simulink library "VehDynaPlayGround"  (R2024b)
settings: Solver=VariableStepAuto  StartTime=0.0  StopTime=10.0  RelTol=1e-3
undefined symbols (not defined in the file or in its folder): A_F, C_af, C_ar, C_d, f, g, h_aero, h_gc, InitialX, InitialY, Iz, lf, lr, m, Nf, Nr, phi, r_stat, r_w, rho, theta, V_wind
libraries: slpidlib x5
(part 2 of 3)

== matlab function VehDynaPlayGround/Vehicle Dynamics/LateralDynamics/LateralDynamicWithNoise/LateralDynamicWithNoise ==
  data: dX output; X input; Vx input; dd input; phi_ref input; NoiseDdy input; NoiseDdpsi input; C_af parameter; C_ar parameter; lf parameter; lr parameter; Iz parameter; m parameter; g parameter
% ******************* Lateral dynamic controller *********************
%*********************************************************************
% Author: L.Arturo Torres-Romero
% Date: 22-10-2020
% BICYCLE MODEL OF LATERAL VEHICLE DYNAMICS
% Based on Rajamani chapter 2.3 page 30 and  in the next publication with
% the controller
% https://www.researchgate.net/publication/340166902_LATERAL_VEHICLE_DYNAMICS_AND_CONTROLLERS_DESIGN
%******************* PARAMETERS DESCRIPTIONS **********************
%******************************************************************
% m: vehicle mass
% g: gravity
% C_af : Cornering  stiffness  of  front  wheels.
% C_ar : Cornering  stiffness  of  rear  wheels.
% lf : distance fron the center of gravity to the front wheel axis.
% lr : distance fron the center of gravity to the rear wheel axis.
% Iz : this is the momentum of inertia of the vehicle respect the z axis.
% phi: is the road bank.
%******************************************************************
%******************* INPUTS DESCRIPTIONS **************************
%******************************************************************
% X:   (column vector)[y;dy;Psi;dPsi] states of the state space of 
%       the system that includes:
%      y  : Radius of the curve that the car is performing.
%      dy : Lateral velocity.
%      Psi  : Is the yaw angle respect to the inertial global system
%      dPsi : Angular velocity of the yaw angle.
% Vx: Logitudinal velocity.

function dX = DynamicBicycleModel2(X,Vx,dd, phi_ref, NoiseDdy, NoiseDdpsi, C_af, C_ar, lf, lr, Iz, m,g) % pd polos deseados
dX = [0;0;0;0];
y = X(1);
dy = X(2);
Psi = X(3);
dPsi = X(4);
phi = phi_ref;

theta_vf = atan((dy + lf*dPsi)/Vx);
theta_vr = atan((dy - lr*dPsi)/Vx);

alpha_f = dd - theta_vf; % lateral slip angle in front tires
alpha_r = -theta_vr; % lateral slip angle in rear tires

dX(1) = X(2);
dX(2) = NoiseDdy + (2*C_af*alpha_f + 2*C_ar*alpha_r)/m + g*sin(phi) - dPsi*Vx;
dX(3) = X(4);
dX(4) = NoiseDdpsi + (2*lf*C_af*alpha_f - 2*lr*C_ar*alpha_r)/Iz;

end

== matlab function VehDynaPlayGround/Control laws/LateralController/SMC_Conventional1 ==
  data: U output size=1; E input; Vx input; C_af parameter; g parameter; C_ar parameter; lf parameter; lr parameter; Iz parameter; m parameter
% ******************* Lateral dynamic controller *********************
%*********************************************************************
% Author: L.Arturo Torres-Romero
% Date: 22-10-2020
% This controller controlls the direction of a car, based in the dynamics
% described  in the next link and using the conventional sliding mode control 
% formulation with the procedure of converting to regular form: 
% https://www.researchgate.net/publication/340166902_LATERAL_VEHICLE_DYNAMICS_AND_CONTROLLERS_DESIGN
%******************* PARAMETERS DESCRIPTIONS **********************
%******************************************************************
% m: vehicle mass
% g: gravity
% C_af : Cornering  stiffness  of  front  wheels.
% C_ar : Cornering  stiffness  of  rear  wheels.
% lf : distance fron the center of gravity to the front wheel axis.
% lr : distance fron the center of gravity to the rear wheel axis.
% Iz : this is the momentum of inertia of the vehicle respect the z axis.
%******************************************************************
%******************* INPUTS DESCRIPTIONS **************************
%******************************************************************
% E:   (column vector)[e1;de1;e2;de2] states of the state space of 
%       the system that includes the errors as follows:
%      e1  : is the lateral position error respect the road.
%      de1 : derivative of e1.
%      e2  : is the yaw angle error with respect the road. 
%      de2 : derivarive of the e2.
% Vx: Logitudinal velocity.

%******************************************************************
% ******************* OUTPUTS DESCRIPTIONS ************************
%******************************************************************
% U: control coutput in radians. Angle of the frontal wheels respect to the
%    longitudinal axis
% isCtrl: when true means that the matrix Mc has full rank, and hence, the
%         system is controllable
%******************************************************************

function U = SMC_ConventionalCtrl(E, Vx, C_af, g, C_ar, lf, lr, Iz, m) % pd polos deseados
X = [0; 0; 0; 0];
X(1) = E(1);
X(2) = E(2);
X(3) = E(3);
X(4) = E(4);
n = 16;
lambda_1 = -1;
lambda_2 = -2;
%**************************************************
%******* Matrix A formulation *********************
A22 = -(2*C_af + 2*C_ar)/(m*Vx);
A23 = (2*C_af + 2*C_ar)/m;
A24 = (-2*C_af*lf + 2*C_ar*lr)/(m*Vx);
A42 = -(2*C_af*lf - 2*C_ar*lr)/(Iz*Vx);
A43 = (2*C_af*lf - 2*C_ar*lr)/Iz;
A44 = -(2*C_af*lf^2 + 2*C_ar*lr^2)/(Iz*Vx);

A = [0 1 0 0;0 A22 A23 A24;0 0 0 1;0 A42 A43 A44];
%**************************************************

%**************************************************
%******* Matrix B1 formulation ********************
B1_2 = 2*C_af/m;
B1_4 = 2*C_af*lf/Iz;

B1 = [0;B1_2;0;B1_4];
%***************************************************

%***************************************************
%******* Matrix B2 formulation *********************
B2_2 = -(2*C_af*lf - 2*C_ar*lr)/(m*Vx) - Vx;
B2_4 = -(2*C_af*lf^2 + 2*C_ar*lr^2)/(Iz*Vx);

B2 = [0;B2_2;0;B2_4];
%***************************************************


%***************************************************
%******* Matrix B3 formulation *********************
B3 = [0;g;0;0];
%***************************************************
x1 = X(1);
x2 = X(2);
x3 = X(3);
x4 = X(4);

%%%%%% this is with S2 = inv(B_2)
% sigma1 = -(lambda_2*x1 - x2 + lambda_2*x3)/B1_2;
% sigma2 = -(lambda_1*x1 - x4 + lambda_1*x3)/B1_4;
% u1 = -(A22*x2 + A23*x3 + A24*x4 - lambda_2*x2 - lambda_2*x4 + B1_2*n*sign(sigma1))/B1_2;
% u2 = -(A42*x2 + A43*x3 + A44*x4 - lambda_1*x2 - lambda_1*x4 + B1_4*n*sign(sigma2))/B1_4;


%%%%%% this is with S2 = eye(2)
sigma1 = -(abs(B1_4)*(lambda_1*x1 - x4 + lambda_1*x3))/B1_4;
sigma2 = -(abs(B1_2)*(lambda_2*x1 - x2 + lambda_2*x3))/B1_2;
u1 = -(A42*x2 + A43*x3 + A44*x4 - lambda_1*x2 - lambda_1*x4 + n*sign(B1_4)*sign(sigma1))/B1_4;
u2 = -(A22*x2 + A23*x3 + A24*x4 - lambda_2*x2 - lambda_2*x4 + n*sign(B1_2)*sign(sigma2))/B1_2;

ctrlVal =  (u2+u1)/2;

U = real(ctrlVal);    



%*****************************************************************************
%******* Live script for help in calculus of the controller ************
% 
% format rational
% syms A B Q R Tr B1_2 B1_4 A22 A23 A24 A42 A43 A44
% A = [0 1 0 0;0 A22 A23 A24;0 0 0 1;0 A42 A43 A44]
% B = [0 0;B1_2 0;0 0;0 B1_4]
% 
% [Q R] = qr(sym(B))
% 
% Tr= flipud(Q') % we need the cero part in the superior part
% rank(Tr)
% 
% B_ = Tr*B
% 
% A_ = Tr*A*inv(Tr)
% 
% % A_ matrix partition
% A_11 = A_(1:2,1:2)
% A_12 = A_(1:2,3:4)
% A_21 = A_(3:4,1:2)
% A_22 = A_(3:4,3:4)
% 
% syms M M11 M12 M21 M22 lambda_1 lambda_2
% M = [M11 M12;M21 M22];
% eqeigen = [lambda_1;lambda_2] == A_11 - A_12*M;
% H = solve(eqeigen,M);
% M_ = [H.M11 H.M12;H.M21 H.M22]
% 
% S2 = eye(2);
% %S2 = inv(B_(3:4,:))
% S = S2*[M_ eye(2)]*Tr;
% disp("surface S: ")
% expand(S)
% 
% syms n sigma_ x1 x2 x3 x4 u1 u2
% X = [x1;x2;x3;x4];
% U = [u1;u2];
% 
% SIGMA = S*X;
% Sigma_1 = simplify(SIGMA(1))
% Sigma_2 = simplify(SIGMA(2))
% 
% eqsolution = -n*sign(sigma_) == S*(A*X + B*U)
% sol1 = solve(eqsolution(1),u2);
% sol2 = solve(eqsolution(2),u1);
% 
% simplify(sol1)
% simplify(sol2)

== matlab function VehDynaPlayGround/Vehicle Dynamics/LateralDynamics/LateralDynamic ==
  data: dX output; X input; Vx input; dd input; C_af parameter; C_ar parameter; lf parameter; lr parameter; Iz parameter; m parameter; g parameter; phi_ref input
% ******************* Lateral dynamic controller *********************
%*********************************************************************
% Author: L.Arturo Torres-Romero
% Date: 22-10-2020
% BICYCLE MODEL OF LATERAL VEHICLE DYNAMICS
% Based on Rajamani chapter 2.3 page 30 and  in the next publication with
% the controller
% https://www.researchgate.net/publication/340166902_LATERAL_VEHICLE_DYNAMICS_AND_CONTROLLERS_DESIGN
%******************* PARAMETERS DESCRIPTIONS **********************
%******************************************************************
% m: vehicle mass
% g: gravity
% C_af : Cornering  stiffness  of  front  wheels.
% C_ar : Cornering  stiffness  of  rear  wheels.
% lf : distance fron the center of gravity to the front wheel axis.
% lr : distance fron the center of gravity to the rear wheel axis.
% Iz : this is the momentum of inertia of the vehicle respect the z axis.
% phi : is the road bank. not used in this model.
%******************************************************************
%******************* INPUTS DESCRIPTIONS **************************
%******************************************************************
% X:   (column vector)[y;dy;Psi;dPsi] states of the state space of 
%       the system that includes:
%      y  : Radius of the curve that the car is performing.
%      dy : Lateral velocity.
%      Psi  : Is the yaw angle respect to the inertial global system
%      dPsi : Angular velocity of the yaw angle.
% Vx: Logitudinal velocity.

function dX = DynamicBicycleModel(X,Vx,dd, C_af, C_ar, lf, lr, Iz, m,g, phi_ref) % pd polos deseados
dX = [0;0;0;0];
y = X(1);
dy = X(2);
Psi = X(3);
dPsi = X(4);
phi = phi_ref;

A22 = -(2*C_af+2*C_ar)/(m*Vx);
A24 = -Vx- (2*C_af*lf-2*C_ar*lr)/(m*Vx);
A42 = -(2*lf*C_af-2*lr*C_ar)/(Iz*Vx);
A44 = -(2*lf^2*C_af + 2*lr^2*C_ar)/(Iz*Vx);

B21 = 2*C_af/m;
B41 = 2*lf*C_af/Iz;

A = [0 1 0 0;0 A22 0 A24;0 0 0 1;0 A42 0 A44];
B = [0;B21;0;B41];

dX= A*X(1:4) + B*dd; 

end

== matlab function VehDynaPlayGround/Model helpers/CoordConvertRotation/MATLAB Function ==
  data: A input; B output; theta input
function B = RotateVector(A, theta)
B = [0;0];
R = [cos(theta) -sin(theta); sin(theta) cos(theta)];

B = R*A;

== matlab function VehDynaPlayGround/Vehicle Dynamics/LateralDynamics/LateralDynamic2 ==
  data: dX output; X input; Vx input; dd input; phi_ref input; C_af parameter; C_ar parameter; lf parameter; lr parameter; Iz parameter; m parameter; g parameter
% ******************* Lateral dynamic controller *********************
%*********************************************************************
% Author: L.Arturo Torres-Romero
% Date: 22-10-2020
% BICYCLE MODEL OF LATERAL VEHICLE DYNAMICS
% Based on Rajamani chapter 2.3 page 30 and  in the next publication with
% the controller
% https://www.researchgate.net/publication/340166902_LATERAL_VEHICLE_DYNAMICS_AND_CONTROLLERS_DESIGN
%******************* PARAMETERS DESCRIPTIONS **********************
%******************************************************************
% m: vehicle mass
% g: gravity
% C_af : Cornering  stiffness  of  front  wheels.
% C_ar : Cornering  stiffness  of  rear  wheels.
% lf : distance fron the center of gravity to the front wheel axis.
% lr : distance fron the center of gravity to the rear wheel axis.
% Iz : this is the momentum of inertia of the vehicle respect the z axis.
% phi: is the road bank.
%******************************************************************
%******************* INPUTS DESCRIPTIONS **************************
%******************************************************************
% X:   (column vector)[y;dy;Psi;dPsi] states of the state space of 
%       the system that includes:
%      y  : Radius of the curve that the car is performing.
%      dy : Lateral velocity.
%      Psi  : Is the yaw angle respect to the inertial global system
%      dPsi : Angular velocity of the yaw angle.
% Vx: Logitudinal velocity.

function dX = DynamicBicycleModel2(X,Vx,dd,phi_ref, C_af, C_ar, lf, lr, Iz, m,g) % pd polos deseados
dX = [0;0;0;0];
y = X(1);
dy = X(2);
Psi = X(3);
dPsi = X(4);

theta_vf = atan((dy + lf*dPsi)/Vx);
theta_vr = atan((dy - lr*dPsi)/Vx);

alpha_f = dd - theta_vf; % lateral slip angle in front tires
alpha_r = -theta_vr; % lateral slip angle in rear tires

dX(1) = X(2);
dX(2) = (2*C_af*alpha_f + 2*C_ar*alpha_r)/m + g*sin(phi_ref) - dPsi*Vx;
dX(3) = X(4);
dX(4) = (2*lf*C_af*alpha_f - 2*lr*C_ar*alpha_r)/Iz;

end

== matlab function VehDynaPlayGround/Electric Actuators/SteeringActuator/BLDC_AngleCtrl/Back EMF ==
  data: X input; Fabc output
function Fabc = fcn(X)
Fabc = [0;0;0];
    theta = mod(X(5),2*pi); %X(4)
    %theta = mod(X,2*pi);
    
    if (0<=theta)&&(theta<(pi/6))
        Fa = (6/pi)*theta;
    elseif ((pi/6)<=theta)&&(theta<(5*pi/6))
        Fa = 1;
    elseif ((5*pi/6<=theta))&&(theta<(7*pi/6))
        Fa = (6/pi)*(pi-theta);
    elseif ((7*pi/6)<=theta)&&(theta<(11*pi/6))
        Fa = -1;
    elseif ((11*pi/6)<=theta)&&(theta<(2*pi))
        Fa = (6/pi)*(theta-2*pi);
    else
        Fa = NaN;
    end
    
    if (0<=theta)&&(theta<(3*pi/6))
        Fb = -1;
    elseif ((3*pi/6)<=theta)&&(theta<(5*pi/6))
        Fb = (6/pi)*(theta-(2*pi)/3);
    elseif ((5*pi/6)<=theta)&&(theta<(9*pi/6))
        Fb = 1;
    elseif ((9*pi/6)<=theta)&&(theta<(11*pi/6))
        Fb = (6/pi)*(-theta+(5*pi)/3);
    elseif ((11*pi/6)<=theta)&&(theta<(2*pi))
        Fb = -1;
    else
        Fb = NaN;
    end
    
    if (0<=theta)&&(theta<(pi/6))
        Fc = 1;
    elseif ((pi/6)<=theta)&&(theta<(3*pi/6))
        Fc = (6/pi)*(pi/3-theta);
    elseif ((3*pi/6)<=theta)&&(theta<(7*pi/6))
        Fc = -1;
    elseif ((7*pi/6)<=theta)&&(theta<(9*pi/6))
        Fc = (6/pi)*(theta-(4*pi)/3);
    elseif ((9*pi/6)<=theta)&&(theta<(2*pi))
        Fc = 1;
    else
        Fc = NaN; 
    end
    
    
%     
     %Fa = sin(theta);
     %Fb = sin(theta - 2*pi/3);
     %Fc = sin(theta + 2*pi/3);
    
    Fabc = [Fa;Fb;Fc];
end

== matlab function VehDynaPlayGround/Electric Actuators/SteeringActuator/BLDC_AngleCtrl/InvParkClarke ==
  data: X_dq input; Y_abc output; theta input
function Y_abc = fcn(X_dq, theta)
X_dq0 = [X_dq; 0];

%inverse Park-Clarke power invariant
iT_PC = sqrt(2/3)*[cos(theta)          -sin(theta)            1/sqrt(2); ...
                  cos(theta-2*pi/3)   -sin(theta-2*pi/3)     1/sqrt(2); ...
                  cos(theta+2*pi/3)   -sin(theta+2*pi/3)     1/sqrt(2)];
%               
              
 %inverse Park-Clarke amplitude invariant
% iT_PC = [cos(theta)          -sin(theta)            1; ...
%          cos(theta-2*pi/3)   -sin(theta-2*pi/3)     1; ...
%          cos(theta+2*pi/3)   -sin(theta+2*pi/3)     1];



Y_abc =iT_PC*X_dq0;
end

== matlab function VehDynaPlayGround/Electric Actuators/SteeringActuator/BLDC_AngleCtrl/ParkClarke ==
  data: X_abc input; Y_dq output; theta input
function Y_dq = fcn(X_abc, theta)

% Park clarke transform eliminating the third element
PC_T = (sqrt(2)/2)*[sqrt(3)*cos(theta)  sin(theta)  -sin(theta) ; ...
                    -sqrt(3)*sin(theta)  cos(theta)  -cos(theta)];

Y_dq =PC_T*X_abc;
end

== matlab function VehDynaPlayGround/Control laws/LateralController/HOSMC_AckermanSuperTwist/HOSMC_AckermanSuperTwis1 ==
  data: U output size=1; E input; Vx input; Mu1 input; C_af parameter; g parameter; C_ar parameter; lf parameter; lr parameter; Iz parameter; m parameter; dMu1 output
% ******************* Lateral dynamic controller *********************
%*********************************************************************
% Author: L.Arturo Torres-Romero
% Date: 22-10-2020
% This controller controlls the direction of a car, based in the dynamics
% described  in the next link and using the conventional sliding mode control 
% formulation with the procedure of converting to regular form: 
% https://www.researchgate.net/publication/340166902_LATERAL_VEHICLE_DYNAMICS_AND_CONTROLLERS_DESIGN
%******************* PARAMETERS DESCRIPTIONS **********************
%******************************************************************
% m: vehicle mass
% g: gravity
% C_af : Cornering  stiffness  of  front  wheels.
% C_ar : Cornering  stiffness  of  rear  wheels.
% lf : distance fron the center of gravity to the front wheel axis.
% lr : distance fron the center of gravity to the rear wheel axis.
% Iz : this is the momentum of inertia of the vehicle respect the z axis.
%******************************************************************
%******************* INPUTS DESCRIPTIONS **************************
%******************************************************************
% E:   (column vector)[e1;de1;e2;de2] states of the state space of 
%       the system that includes the errors as follows:
%      e1  : is the lateral position error respect the road.
%      de1 : derivative of e1.
%      e2  : is the yaw angle error with respect the road. 
%      de2 : derivarive of the e2.
% Vx: Logitudinal velocity.

%******************************************************************
% ******************* OUTPUTS DESCRIPTIONS ************************
%******************************************************************
% U: control coutput in radians. Angle of the frontal wheels respect to the
%    longitudinal axis
% isCtrl: when true means that the matrix Mc has full rank, and hence, the
%         system is controllable
%******************************************************************

function [U, dMu1] = SMC_AckermanSuperTwistingCtrl(E, Vx, Mu1,C_af, g, C_ar, lf, lr, Iz, m) % pd polos deseados
X = [0; 0; 0; 0];
X(1) = E(1);
X(2) = E(2);
X(3) = E(3);
X(4) = E(4);
%**************************************************
%******* Matrix A formulation *********************
A22 = -(2*C_af + 2*C_ar)/(m*Vx);
A23 = (2*C_af + 2*C_ar)/m;
A24 = (-2*C_af*lf + 2*C_ar*lr)/(m*Vx);
A42 = -(2*C_af*lf - 2*C_ar*lr)/(Iz*Vx);
A43 = (2*C_af*lf - 2*C_ar*lr)/Iz;
A44 = -(2*C_af*lf^2 + 2*C_ar*lr^2)/(Iz*Vx);

A = [0 1 0 0;0 A22 A23 A24;0 0 0 1;0 A42 A43 A44];
%**************************************************

%**************************************************
%******* Matrix B1 formulation ********************
B1_2 = 2*C_af/m;
B1_4 = 2*C_af*lf/Iz;

B1 = [0;B1_2;0;B1_4];
%***************************************************

%***************************************************
%******* Matrix B2 formulation *********************
B2_2 = -(2*C_af*lf - 2*C_ar*lr)/(m*Vx) - Vx;
B2_4 = -(2*C_af*lf^2 + 2*C_ar*lr^2)/(Iz*Vx);

B2 = [0;B2_2;0;B2_4];
%***************************************************


%***************************************************
%******* Matrix B3 formulation *********************
B3 = [0;g;0;0];
%***************************************************


%***************************************************
%******* Verification of controllability and output 
% calculation of the controller
%**************************************************
d_k = 0;
Mc = [B1 A*B1 A^2*B1 A^3*B1];
rankVal = rank(Mc);
    if rankVal < size(A,1)
        %disp('Not completely state controllable');
        isCtrl = 0;
        d_k = 0;
    else
        %disp('Completely state controllable');
        isCtrl = 1;
        % Pole placement
        %Pd =[-5-3i -5+3i -7 -10];
        Pd =[-5-5i -5+5i -7 -10];

        H = (A- Pd(1)*eye(4)) * (A- Pd(2)*eye(4)) * (A- Pd(3)*eye(4)) * (A- Pd(4)*eye(4));

        %ackerman formula
        K = [0 0 0 1]*Mc^-1*H;
        d_k = -K*X;  
    end

%*********** Controller parameters **************
k_smc = 100;   %10
sigma = 40;    %60
gamma1 = 1;
gamma2 = 1;
gamma = [0 gamma1 0 gamma2];

h_c = gamma*[0;3;0;3];
g_c = gamma*B1;
q = 0.3;

UM = abs(h_c/g_c)/q;

%***********************************************
e_c = gamma*[0; X(1);0;X(3)];
d_u = (-1/(gamma*B1))*(sigma*sqrt(abs(e_c))*sign(e_c) + Mu1);

if abs(Mu1) > UM 
   dMu1 = -Mu1;
else
   dMu1 = -k_smc*sign(e_c); 
end

ctrlVal = d_k + d_u;

U = real(ctrlVal);

== matlab function VehDynaPlayGround/Control laws/LateralController/SMC_Conventional2 ==
  data: U output size=1; E input; Vx input; dPsi_des input; C_af parameter; g parameter; C_ar parameter; lf parameter; lr parameter; Iz parameter; m parameter; phi_ref input

% ******************* Lateral dynamic controller *********************
%*********************************************************************
% Author: L.Arturo Torres-Romero
% Date: 22-10-2020
% This controller controlls the direction of a car, based in the dynamics
% described  in the next link and using the conventional sliding mode control 
% formulation with the procedure of converting to regular form: 
% https://www.researchgate.net/publication/340166902_LATERAL_VEHICLE_DYNAMICS_AND_CONTROLLERS_DESIGN
%******************* PARAMETERS DESCRIPTIONS **********************
%******************************************************************
% m: vehicle mass
% g: gravity
% C_af : Cornering  stiffness  of  front  wheels.
% C_ar : Cornering  stiffness  of  rear  wheels.
% lf : distance fron the center of gravity to the front wheel axis.
% lr : distance fron the center of gravity to the rear wheel axis.
% Iz : this is the momentum of inertia of the vehicle respect the z axis.
%******************************************************************
%******************* INPUTS DESCRIPTIONS **************************
%******************************************************************
% E:   (column vector)[e1;de1;e2;de2] states of the state space of 
%       the system that includes the errors as follows:
%      e1  : is the lateral position error respect the road.
%      de1 : derivative of e1.
%      e2  : is the yaw angle error with respect the road. 
%      de2 : derivarive of the e2.
% Vx: Logitudinal velocity.

%******************************************************************
% ******************* OUTPUTS DESCRIPTIONS ************************
%******************************************************************
% U: control coutput in radians. Angle of the frontal wheels respect to the
%    longitudinal axis
% isCtrl: when true means that the matrix Mc has full rank, and hence, the
%         system is controllable
%******************************************************************

function U = SMC_ConventionalCtr2(E, Vx, dPsi_des,C_af, g, C_ar, lf, lr, Iz, m, phi_ref) % pd polos deseados
J = [0; 0; 0; 0];
J(1) = E(3);
J(2) = E(4);
J(3) = E(1);
J(4) = E(2);
phi = phi_ref;
%**************************************************
%******* Matrix A formulation *********************
A22 = -(2*C_af + 2*C_ar)/(m*Vx);
A23 = (2*C_af + 2*C_ar)/m;
A24 = (-2*C_af*lf + 2*C_ar*lr)/(m*Vx);
A42 = -(2*C_af*lf - 2*C_ar*lr)/(Iz*Vx);
A43 = (2*C_af*lf - 2*C_ar*lr)/Iz;
A44 = -(2*C_af*lf^2 + 2*C_ar*lr^2)/(Iz*Vx);

%A = [0 1 0 0;0 A22 A23 A24;0 0 0 1;0 A42 A43 A44];
A = [0 0 0 1;0 A42 A43 A44;0 1 0 0;0 A22 A23 A24];

%**************************************************

%**************************************************
%******* Matrix B1 formulation ********************
B1_2 = 2*C_af/m;
B1_4 = 2*C_af*lf/Iz;

%B1 = [0;B1_2;0;B1_4];
B1 = [0;B1_4;0;B1_2];
%***************************************************

%***************************************************
%******* Matrix B2 formulation *********************
B2_2 = -(2*C_af*lf - 2*C_ar*lr)/(m*Vx) - Vx;
B2_4 = -(2*C_af*lf^2 + 2*C_ar*lr^2)/(Iz*Vx);

B2 = [0;B2_4;0;B2_2];
%***************************************************


%***************************************************
%******* Matrix B3 formulation *********************
B3 = [0;g;0;0];
%***************************************************

l1 = (A24 - Vx)*dPsi_des +g*sin(phi);
l2 = A44*dPsi_des;
L = [0;l2;0;l1];

C = [B1 A*B1 A^2*B1 A^3*B1]; % controllability matrix
Cinv = inv(C);
q = Cinv(4,:);
P = [q;q*A;q*A^2;q*A^3];
Tr = P;

X = Tr*J;

%%%%%%%%%%%%%%%%%%%%%%%%%%%%% SMC settings %%%%%%%%%%%%%%%%%%%%%%%%%%%%%%%
n1 = 140000;
lambda_1 = -2;
lambda_2 = -7;
lambda_3 = -3;

S = [(1000000*lambda_1*lambda_2*lambda_3)/(A23*B1_4 - A43*B1_2), (1000000*(A23^2*B1_4^3 + A43^2*B1_2^2*B1_4 + A22*A23*A24*B1_4^3 - A42*A43*A44*B1_2^3 - 2*A23*A43*B1_2*B1_4^2 - A43*A44*B1_2^3*lambda_1 - A43*A44*B1_2^3*lambda_2 - A43*A44*B1_2^3*lambda_3 - A22*A23*A44*B1_2*B1_4^2 - A22*A24*A43*B1_2*B1_4^2 - A23*A24*A42*B1_2*B1_4^2 + A22*A43*A44*B1_2^2*B1_4 + A23*A42*A44*B1_2^2*B1_4 + A24*A42*A43*B1_2^2*B1_4 - A23*A24*B1_2*B1_4^2*lambda_1 - A23*A24*B1_2*B1_4^2*lambda_2 - A23*A24*B1_2*B1_4^2*lambda_3 + A23*A44*B1_2^2*B1_4*lambda_1 + A24*A43*B1_2^2*B1_4*lambda_1 + A23*A44*B1_2^2*B1_4*lambda_2 + A24*A43*B1_2^2*B1_4*lambda_2 + A23*A44*B1_2^2*B1_4*lambda_3 + A24*A43*B1_2^2*B1_4*lambda_3 - A23*B1_2*B1_4^2*lambda_1*lambda_2 - A23*B1_2*B1_4^2*lambda_1*lambda_3 - A23*B1_2*B1_4^2*lambda_2*lambda_3 + A43*B1_2^2*B1_4*lambda_1*lambda_2 + A43*B1_2^2*B1_4*lambda_1*lambda_3 + A43*B1_2^2*B1_4*lambda_2*lambda_3 - A44*B1_2^3*lambda_1*lambda_2*lambda_3 + A22*B1_2*B1_4^2*lambda_1*lambda_2*lambda_3 + A24*B1_2^2*B1_4*lambda_1*lambda_2*lambda_3 - A42*B1_2^2*B1_4*lambda_1*lambda_2*lambda_3))/((A23*B1_4 - A43*B1_2)*(A24^2*B1_2*B1_4^2 - 2*A24*A44*B1_2^2*B1_4 - A42*A24*B1_2*B1_4^2 + A22*A24*B1_4^3 + A44^2*B1_2^3 + A42*A44*B1_2^2*B1_4 - A22*A44*B1_2*B1_4^2 - A43*B1_2*B1_4^2 + A23*B1_4^3)), (1000000*(A23^2*B1_4^3*lambda_1 + A23^2*B1_4^3*lambda_2 + A23^2*B1_4^3*lambda_3 + A23^2*A24*B1_4^3 - A43^2*A44*B1_2^3 + A24*A43^2*B1_2^2*B1_4 - A23^2*A44*B1_2*B1_4^2 + A43^2*B1_2^2*B1_4*lambda_1 + A43^2*B1_2^2*B1_4*lambda_2 + A43^2*B1_2^2*B1_4*lambda_3 - 2*A23*A24*A43*B1_2*B1_4^2 + 2*A23*A43*A44*B1_2^2*B1_4 - 2*A23*A43*B1_2*B1_4^2*lambda_1 - 2*A23*A43*B1_2*B1_4^2*lambda_2 - 2*A23*A43*B1_2*B1_4^2*lambda_3 - A22*A23*B1_4^3*lambda_1*lambda_2 - A22*A23*B1_4^3*lambda_1*lambda_3 - A22*A23*B1_4^3*lambda_2*lambda_3 - A43*A44*B1_2^3*lambda_1*lambda_2 - A43*A44*B1_2^3*lambda_1*lambda_3 - A43*A44*B1_2^3*lambda_2*lambda_3 + A22^2*B1_4^3*lambda_1*lambda_2*lambda_3 + A42^2*B1_2^2*B1_4*lambda_1*lambda_2*lambda_3 - A23*A24*B1_2*B1_4^2*lambda_1*lambda_2 - A23*A24*B1_2*B1_4^2*lambda_1*lambda_3 - A23*A24*B1_2*B1_4^2*lambda_2*lambda_3 + A22*A43*B1_2*B1_4^2*lambda_1*lambda_2 + A23*A42*B1_2*B1_4^2*lambda_1*lambda_2 + A22*A43*B1_2*B1_4^2*lambda_1*lambda_3 + A23*A42*B1_2*B1_4^2*lambda_1*lambda_3 + A22*A43*B1_2*B1_4^2*lambda_2*lambda_3 + A23*A42*B1_2*B1_4^2*lambda_2*lambda_3 + A23*A44*B1_2^2*B1_4*lambda_1*lambda_2 + A24*A43*B1_2^2*B1_4*lambda_1*lambda_2 + A23*A44*B1_2^2*B1_4*lambda_1*lambda_3 + A24*A43*B1_2^2*B1_4*lambda_1*lambda_3 + A23*A44*B1_2^2*B1_4*lambda_2*lambda_3 + A24*A43*B1_2^2*B1_4*lambda_2*lambda_3 - A42*A43*B1_2^2*B1_4*lambda_1*lambda_2 - A42*A43*B1_2^2*B1_4*lambda_1*lambda_3 - A42*A43*B1_2^2*B1_4*lambda_2*lambda_3 + A42*A44*B1_2^3*lambda_1*lambda_2*lambda_3 - A23*B1_2*B1_4^2*lambda_1*lambda_2*lambda_3 + A43*B1_2^2*B1_4*lambda_1*lambda_2*lambda_3 + A22*A24*B1_2*B1_4^2*lambda_1*lambda_2*lambda_3 - 2*A22*A42*B1_2*B1_4^2*lambda_1*lambda_2*lambda_3 - A22*A44*B1_2^2*B1_4*lambda_1*lambda_2*lambda_3 - A24*A42*B1_2^2*B1_4*lambda_1*lambda_2*lambda_3))/((A23*B1_4 - A43*B1_2)*(A24^2*B1_2*B1_4^2 - 2*A24*A44*B1_2^2*B1_4 - A42*A24*B1_2*B1_4^2 + A22*A24*B1_4^3 + A44^2*B1_2^3 + A42*A44*B1_2^2*B1_4 - A22*A44*B1_2*B1_4^2 - A43*B1_2*B1_4^2 + A23*B1_4^3)), (1000000*(A23*A24^2*B1_4^3 - A43*A44^2*B1_2^3 + A23*B1_4^3*lambda_1*lambda_2 + A23*B1_4^3*lambda_1*lambda_3 + A23*B1_4^3*lambda_2*lambda_3 + A23*A44^2*B1_2^2*B1_4 - A24^2*A43*B1_2*B1_4^2 + A23*A24*B1_4^3*lambda_1 + A23*A24*B1_4^3*lambda_2 + A23*A24*B1_4^3*lambda_3 - 2*A23*A24*A44*B1_2*B1_4^2 + 2*A24*A43*A44*B1_2^2*B1_4 - A23*A44*B1_2*B1_4^2*lambda_1 - A24*A43*B1_2*B1_4^2*lambda_1 - A23*A44*B1_2*B1_4^2*lambda_2 - A24*A43*B1_2*B1_4^2*lambda_2 - A23*A44*B1_2*B1_4^2*lambda_3 - A24*A43*B1_2*B1_4^2*lambda_3 + A43*A44*B1_2^2*B1_4*lambda_1 + A43*A44*B1_2^2*B1_4*lambda_2 + A43*A44*B1_2^2*B1_4*lambda_3 - A43*B1_2*B1_4^2*lambda_1*lambda_2 - A43*B1_2*B1_4^2*lambda_1*lambda_3 - A43*B1_2*B1_4^2*lambda_2*lambda_3 - A22*B1_4^3*lambda_1*lambda_2*lambda_3 - A24*B1_2*B1_4^2*lambda_1*lambda_2*lambda_3 + A42*B1_2*B1_4^2*lambda_1*lambda_2*lambda_3 + A44*B1_2^2*B1_4*lambda_1*lambda_2*lambda_3))/((A23*B1_4 - A43*B1_2)*(A24^2*B1_2*B1_4^2 - 2*A24*A44*B1_2^2*B1_4 - A42*A24*B1_2*B1_4^2 + A22*A24*B1_4^3 + A44^2*B1_2^3 + A42*A44*B1_2^2*B1_4 - A22*A44*B1_2*B1_4^2 - A43*B1_2*B1_4^2 + A23*B1_4^3))];

%%%%%%%%%%%%%%%%%%%%%%%%%%%%%%%%%%%%%%%%%%%%%%%%%%%%%%%%%%%%%%%%%%%%%%%%%%%%

sigma1 = S*X;
ctrlVal = -(S*B1)\(n1*sign(sigma1)+ S*A*X +S*L);
U = real(ctrlVal);    



%*****************************************************************************
%******* Live script for help in calculus of the controller ************
% 
% format rational
% syms A B Q R Tr B1_2 B1_4 A22 A23 A24 A42 A43 A44 delta x1 x2 x3 x4 l1 l2
% 
% % X  = [x1;x2;x3;x4]
% % A  = [0 1 0 0;0 A22 A23 A24;0 0 0 1;0 A42 A43 A44]
% % B1 = [0;B1_2;0;B1_4]
% % L  = [0;l1;0;l2]
% 
% X  = [x3;x4;x1;x2]
% A  = [0 0 0 1;0 A42 A43 A44;0 1 0 0;0 A22 A23 A24]
% B1 = [0;B1_4;0;B1_2]
% L  = [0;l2;0;l1]
% 
% %%%%%%%%%%%%%%%% Transform (Tr) with ackerman form %%%%%%%%%%%%%%%%
% % C = [B1 A*B1 A^2*B1 A^3*B1] % controllability matrix
% % tmp1 = [0 0 0 1]/C;
% % Tr=[tmp1;tmp1*A;tmp1*A^2;tmp1*A^3] % state transformation
% % disp("tmp1")
% % size(tmp1)
% % disp("tmp1*A")
% % size(tmp1*A)
% % disp("tmp1*A^2")
% % size(tmp1*A^2)
% % disp("tmp1*A^3")
% % size(tmp1*A^3)
% % disp("C:")
% % size(C)
% % disp("tmp1:")
% % size(tmp1)
% % disp("Tr:")
% % size(Tr)
% %%%%%%%%%%%%%%%%%%%%%%%%%%%%%%%%%%%%%%%%%%%%%%%%%%%%%%%%%%%%%%%%%
% 
% %%%%%%%%%%%% Transform (Tr) with Utkin apprach %%%%%%%%%%%%%%%%%%
% % B_1 = [0;0;B1_4];
% % B_2 = B1_2;
% % 
% % a = eye(3)
% % b = -B_1*(B_2^(-1))
% % c = [0 0 0]
% % d = B_2^(-1)
% % 
% % Tr = [a b;c d];
% %%%%%%%%%%%%%%%%%%%%%%%%%%%%%%%%%%%%%%%%%%%%%%%%%%%%%%%%%%%%%%%%%%
% 
% 
% %%%%%%%%%%%%%%%% Transform (Tr) with linear system controller form %%%%%%%%%%%%%%%%
% C = [B1 A*B1 A^2*B1 A^3*B1] % controllability matrix
% Cinv = inv(C)
% q = Cinv(4,:)
% P = [q;q*A;q*A^2;q*A^3]
% Tr = P
% %%%%%%%%%%%%%%%%%%%%%%%%%%%%%%%%%%%%%%%%%%%%%%%%%%%%%%%%%%
% 
% A_ = simplify(Tr*A/Tr)
% B_ = simplify(Tr*B1)
% 
% A_11 = A_(1:3,1:3);
% A_12 = A_(1:3,4);
% 
% syms s1 s2 s3 lambda lambda_1 lambda_2 lambda_3 S2
% 
% %find paramters given eigenvalues
% S = [s1 s2 s3];
% eqeigen = det(lambda*eye(3) - (A_11 - A_12*S));
% eqeigen = simplify(eqeigen);
% eqeigen = collect(eqeigen,lambda);
% polyCoef = coeffs(eqeigen, lambda);
% polyCoef = fliplr(polyCoef)
% %%%%%%%%%%%%%%%
% % desired polinomial characteristic
% desiredPoly = (lambda + lambda_1)*(lambda + lambda_2)*(lambda + lambda_3);
% desiredPoly = collect(desiredPoly);
% desiredCoefs = coeffs(desiredPoly, lambda);
% desiredCoefs = fliplr(desiredCoefs)
% 
% eq1 = desiredCoefs(1) == polyCoef(1);
% eq2 = desiredCoefs(2) == polyCoef(2);
% eq3 = desiredCoefs(3) == polyCoef(3);
% eq4 = desiredCoefs(4) == polyCoef(4);
% 
% system1 = [eq2;eq3;eq4];
% sol = solve(system1,[s1 s2 s3]);
% S_ = [sol.s1 sol.s2 sol.s3]
% 
% %test eigen values:
% charEq1 = subs(eqeigen,s1,sol.s1);
% charEq2 = subs(charEq1,s2,sol.s2);
% charEq3 = subs(charEq2,s3,sol.s3)
% tf = isAlways(charEq3==desiredPoly)
% 
% S2 = 1000000;
% S = S2*[S_ 1]*Tr;
% %S = [S_ 1]*Tr;
% disp("!!!!!!!!surface S: ")
% simplify(S)
% 
% 
% syms n sigma1 x1 x2 x3 x4 u1 u2 n1 n2 
% X = [x1;x2;x3;x4];
% U = u1;
% 
% SIGMA = S*X;
% 
% % rewriting to the original forms %%%%%%%%%%%%%%%
% X  = [x1;x2;x3;x4]
% A  = [0 1 0 0;0 A22 A23 A24;0 0 0 1;0 A42 A43 A44]
% B1 = [0;B1_2;0;B1_4]
% %%%%%%%%%%%%%%%%%%%%%%%%%%%%%%%%%%%%%%%%%%%%%%%
% 
% 
% disp("!!!!! Sliding function sigma_1: ")
% Sigma_1 = simplify(SIGMA);
% Sigma_1 = collect(Sigma_1,[x1;x2;x3;x4])
% 
% eqsolution = -n1*sign(sigma1) == S*(A*X + B1*U +L);
% sol1 = solve(eqsolution,u1);
% 
% disp("!!!!! final control u: ")
% finalControl = simplify(sol1);
% finalControl = collect(finalControl,[x1;x2;x3;x4])
% 
% 
% U = -inv(S*B1)*(n1*sign(sigma1)+ S*A*X +S*L)
% 
% isAlways(finalControl==U)

== matlab function VehDynaPlayGround/Tires/Tyre ModelV1/MagicFormula ==
  data: X input; Y output; F_zf input
%BASED ON
%Massimo Guiggiani, The Science of Vehicle Dynamics, Pisa, Italy, Springer Netherlands, 2014.
%Chapter 2.12
%The values of the MF were obtained from the graph in fig. 2.22
function Y = XTireForce(X, F_zf) 
% B stiffness factor
% C shape factor
% D peak value
% E curvature factor
% Sh horizontal shift
% Sv vertical shift

Sh = 0;% Sh horizontal shift
Sv = 0; %vertical shift

D = 3; % ym, maximum value Experimental from graph
C = 1.5;
B = 20;
E = 0;

x = X-Sh;
gamma = C*atan(B*x-E*(B*x-atan(B*x)));
y = F_zf*D*sin(gamma);
Y = (y - Sv);

== matlab function VehDynaPlayGround/Control laws/LateralController/HOSMC_BlocksSuperTwisting/HOSMC_SuperTwisting ==
  data: U output size=1; E input; Vx input; dPsi_des input; phi_ref input; v input; C_af parameter; g parameter; C_ar parameter; lf parameter; lr parameter; Iz parameter; m parameter; dv output; d_u output
% ******************* Lateral dynamic controller *********************

%*********************************************************************
% Author: L.Arturo Torres-Romero
% Date: 22-10-2020
% This controller controlls the direction of a car, based in the dynamics
% described  in the next link and using the conventional sliding mode control 
% formulation with the procedure of converting to regular form: 
% https://www.researchgate.net/publication/340166902_LATERAL_VEHICLE_DYNAMICS_AND_CONTROLLERS_DESIGN
%******************* PARAMETERS DESCRIPTIONS **********************
%******************************************************************
% m: vehicle mass
% g: gravity
% C_af : Cornering  stiffness  of  front  wheels.
% C_ar : Cornering  stiffness  of  rear  wheels.
% lf : distance fron the center of gravity to the front wheel axis.
% lr : distance fron the center of gravity to the rear wheel axis.
% Iz : this is the momentum of inertia of the vehicle respect the z axis.
%******************************************************************
%******************* INPUTS DESCRIPTIONS **************************
%******************************************************************
% E:   (column vector)[e1;de1;e2;de2] states of the state space of 
%       the system that includes the errors as follows:
%      e1  : is the lateral position error respect the road.
%      de1 : derivative of e1.
%      e2  : is the yaw angle error with respect the road. 
%      de2 : derivarive of the e2.
% Vx: Logitudinal velocity.

%******************************************************************
% ******************* OUTPUTS DESCRIPTIONS ************************
%******************************************************************
% U: control coutput in radians. Angle of the frontal wheels respect to the
%    longitudinal axis
% isCtrl: when true means that the matrix Mc has full rank, and hence, the
%         system is controllable
%******************************************************************

function [U, dv,d_u] = HOSMC_SuperTwistingCtrl(E, Vx,dPsi_des, phi_ref, v,C_af, g, C_ar, lf, lr, Iz, m) % pd polos deseados
Y1 = [0;0];
Y2 = [0;0];

Y1 = [E(1);E(3)];
Y2 = [E(2);E(4)];
e = [E(2);E(3);E(4)];
phi = phi_ref;

%**************************************************
%******* Matrix A formulation *********************
A22 = -(2*C_af + 2*C_ar)/(m*Vx);
A23 = (2*C_af + 2*C_ar)/m;
A24 = (-2*C_af*lf + 2*C_ar*lr)/(m*Vx);
A42 = -(2*C_af*lf - 2*C_ar*lr)/(Iz*Vx);
A43 = (2*C_af*lf - 2*C_ar*lr)/Iz;
A44 = -(2*C_af*lf^2 + 2*C_ar*lr^2)/(Iz*Vx);

A = [A22 A23 A24;A42 A43 A44];

%**************************************************
%******* Matrix B1 formulation ********************
B1_2 = 2*C_af/m;
B1_4 = 2*C_af*lf/Iz;

B1 = [B1_2;B1_4];
%***************************************************

%***************************************************
%******* Matrix L formulation *********************
l1 = (A24 - Vx)*dPsi_des +g*sin(phi);
l2 = A44*dPsi_des;
L = [l1;l2];

%***************************************************

%%
%%%%%%%%%%%%%% SUPER TWISTING 1 %%%%%%%%%%%%%%%%%
% %*********** Controller parameters **************
k1 = 7;%6;      %7   18
k2 = 18;%8;
%sigma = 10;    %60   10
gamma1 = 1;
gamma2 = 0.9;
gamma = [gamma1 gamma2];
%***************************************
h_c = abs(gamma*[0.8;0.4]);
g_c = abs(gamma*B1);
U_M = pi/16;

q = abs(h_c/g_c)/U_M + 0.01;
C = abs(h_c)+ 0.5;
k_v = C/(gamma*B1) + 3; %k_v = C/(gamma*B1) + 0.5;

k_u = sqrt(2/(gamma*B1*k_v - C));
k_u = k_u*(gamma*B1*k_v + C)*(1+q);
k_u = k_u/((gamma*B1)*(1-q)) + 1; %k_u = k_u/((gamma*B1)*(1-q)) + 0.8;



%***********************************************
e_b = -gamma*(k1*Y1+Y2);
d_k = (1/(gamma*B1))*(k2*e_b-gamma*(k1*Y2+A*e+L));
s = e_b;%(1/(gamma*B1))*e_b;

d_u = -(1/(gamma*B1))*(k_u*sqrt(abs(s))*sign(s) + v);

if abs(d_u) > U_M 
   dv = -d_u;
else
   dv = -k_v*sign(s); 
end

%%

%ctrlVal = d_k;
ctrlVal = d_k + d_u;
U = real(ctrlVal);

== matlab function VehDynaPlayGround/Control laws/LateralController/HOSMC_RegularFormSuperTwist/HOSMC_RegularFormSuperTwist ==
  data: U output size=1; E input; Vx input; dPsi_des input; Mu1 input; C_af parameter; g parameter; C_ar parameter; lf parameter; lr parameter; Iz parameter; m parameter; dMu1 output; phi parameter
% ******************* Lateral dynamic controller *********************

%*********************************************************************
% Author: L.Arturo Torres-Romero
% Date: 22-10-2020
% This controller controlls the direction of a car, based in the dynamics
% described  in the next link and using the conventional sliding mode control 
% formulation with the procedure of converting to regular form: 
% https://www.researchgate.net/publication/340166902_LATERAL_VEHICLE_DYNAMICS_AND_CONTROLLERS_DESIGN
%******************* PARAMETERS DESCRIPTIONS **********************
%******************************************************************
% m: vehicle mass
% g: gravity
% C_af : Cornering  stiffness  of  front  wheels.
% C_ar : Cornering  stiffness  of  rear  wheels.
% lf : distance fron the center of gravity to the front wheel axis.
% lr : distance fron the center of gravity to the rear wheel axis.
% Iz : this is the momentum of inertia of the vehicle respect the z axis.
%******************************************************************
%******************* INPUTS DESCRIPTIONS **************************
%******************************************************************
% E:   (column vector)[e1;de1;e2;de2] states of the state space of 
%       the system that includes the errors as follows:
%      e1  : is the lateral position error respect the road.
%      de1 : derivative of e1.
%      e2  : is the yaw angle error with respect the road. 
%      de2 : derivarive of the e2.
% Vx: Logitudinal velocity.

%******************************************************************
% ******************* OUTPUTS DESCRIPTIONS ************************
%******************************************************************
% U: control coutput in radians. Angle of the frontal wheels respect to the
%    longitudinal axis
% isCtrl: when true means that the matrix Mc has full rank, and hence, the
%         system is controllable
%******************************************************************

function [U, dMu1] = HOSMC_RegularFormSuperTwistCtrl(E, Vx,dPsi_des, Mu1,C_af, g, C_ar, lf, lr, Iz, m,phi) % pd polos deseados
J = [0; 0; 0; 0];
J(1) = E(3);
J(2) = E(4);
J(3) = E(1);
J(4) = E(2);

%**************************************************
%******* Matrix A formulation *********************
A22 = -(2*C_af + 2*C_ar)/(m*Vx);
A23 = (2*C_af + 2*C_ar)/m;
A24 = (-2*C_af*lf + 2*C_ar*lr)/(m*Vx);
A42 = -(2*C_af*lf - 2*C_ar*lr)/(Iz*Vx);
A43 = (2*C_af*lf - 2*C_ar*lr)/Iz;
A44 = -(2*C_af*lf^2 + 2*C_ar*lr^2)/(Iz*Vx);

%A = [0 1 0 0;0 A22 A23 A24;0 0 0 1;0 A42 A43 A44];
A = [0 0 0 1;0 A42 A43 A44;0 1 0 0;0 A22 A23 A24];

%**************************************************

%**************************************************
%******* Matrix B1 formulation ********************
B1_2 = 2*C_af/m;
B1_4 = 2*C_af*lf/Iz;

%B1 = [0;B1_2;0;B1_4];
B1 = [0;B1_4;0;B1_2];
%***************************************************

%***************************************************
%******* Matrix B2 formulation *********************
B2_2 = -(2*C_af*lf - 2*C_ar*lr)/(m*Vx) - Vx;
B2_4 = -(2*C_af*lf^2 + 2*C_ar*lr^2)/(Iz*Vx);

B2 = [0;B2_4;0;B2_2];
%***************************************************


%***************************************************
%******* Matrix B3 formulation *********************
B3 = [0;g;0;0];
%***************************************************

l1 = (A24 - Vx)*dPsi_des +g*sin(phi);
l2 = A44*dPsi_des;
L = [0;l2;0;l1];

C = [B1 A*B1 A^2*B1 A^3*B1]; % controllability matrix
Cinv = inv(C);
q = Cinv(4,:);
P = [q;q*A;q*A^2;q*A^3];
Tr = P;

X = Tr*J;

%%%%%%%%%%%%%%%%%%%%%%%%%%%%% SMC settings %%%%%%%%%%%%%%%%%%%%%%%%%%%%%%%
n1 = 1;%140000;
lambda_1 = -2;
lambda_2 = -7;
lambda_3 = -3;

S = [(1000000*lambda_1*lambda_2*lambda_3)/(A23*B1_4 - A43*B1_2), (1000000*(A23^2*B1_4^3 + A43^2*B1_2^2*B1_4 + A22*A23*A24*B1_4^3 - A42*A43*A44*B1_2^3 - 2*A23*A43*B1_2*B1_4^2 - A43*A44*B1_2^3*lambda_1 - A43*A44*B1_2^3*lambda_2 - A43*A44*B1_2^3*lambda_3 - A22*A23*A44*B1_2*B1_4^2 - A22*A24*A43*B1_2*B1_4^2 - A23*A24*A42*B1_2*B1_4^2 + A22*A43*A44*B1_2^2*B1_4 + A23*A42*A44*B1_2^2*B1_4 + A24*A42*A43*B1_2^2*B1_4 - A23*A24*B1_2*B1_4^2*lambda_1 - A23*A24*B1_2*B1_4^2*lambda_2 - A23*A24*B1_2*B1_4^2*lambda_3 + A23*A44*B1_2^2*B1_4*lambda_1 + A24*A43*B1_2^2*B1_4*lambda_1 + A23*A44*B1_2^2*B1_4*lambda_2 + A24*A43*B1_2^2*B1_4*lambda_2 + A23*A44*B1_2^2*B1_4*lambda_3 + A24*A43*B1_2^2*B1_4*lambda_3 - A23*B1_2*B1_4^2*lambda_1*lambda_2 - A23*B1_2*B1_4^2*lambda_1*lambda_3 - A23*B1_2*B1_4^2*lambda_2*lambda_3 + A43*B1_2^2*B1_4*lambda_1*lambda_2 + A43*B1_2^2*B1_4*lambda_1*lambda_3 + A43*B1_2^2*B1_4*lambda_2*lambda_3 - A44*B1_2^3*lambda_1*lambda_2*lambda_3 + A22*B1_2*B1_4^2*lambda_1*lambda_2*lambda_3 + A24*B1_2^2*B1_4*lambda_1*lambda_2*lambda_3 - A42*B1_2^2*B1_4*lambda_1*lambda_2*lambda_3))/((A23*B1_4 - A43*B1_2)*(A24^2*B1_2*B1_4^2 - 2*A24*A44*B1_2^2*B1_4 - A42*A24*B1_2*B1_4^2 + A22*A24*B1_4^3 + A44^2*B1_2^3 + A42*A44*B1_2^2*B1_4 - A22*A44*B1_2*B1_4^2 - A43*B1_2*B1_4^2 + A23*B1_4^3)), (1000000*(A23^2*B1_4^3*lambda_1 + A23^2*B1_4^3*lambda_2 + A23^2*B1_4^3*lambda_3 + A23^2*A24*B1_4^3 - A43^2*A44*B1_2^3 + A24*A43^2*B1_2^2*B1_4 - A23^2*A44*B1_2*B1_4^2 + A43^2*B1_2^2*B1_4*lambda_1 + A43^2*B1_2^2*B1_4*lambda_2 + A43^2*B1_2^2*B1_4*lambda_3 - 2*A23*A24*A43*B1_2*B1_4^2 + 2*A23*A43*A44*B1_2^2*B1_4 - 2*A23*A43*B1_2*B1_4^2*lambda_1 - 2*A23*A43*B1_2*B1_4^2*lambda_2 - 2*A23*A43*B1_2*B1_4^2*lambda_3 - A22*A23*B1_4^3*lambda_1*lambda_2 - A22*A23*B1_4^3*lambda_1*lambda_3 - A22*A23*B1_4^3*lambda_2*lambda_3 - A43*A44*B1_2^3*lambda_1*lambda_2 - A43*A44*B1_2^3*lambda_1*lambda_3 - A43*A44*B1_2^3*lambda_2*lambda_3 + A22^2*B1_4^3*lambda_1*lambda_2*lambda_3 + A42^2*B1_2^2*B1_4*lambda_1*lambda_2*lambda_3 - A23*A24*B1_2*B1_4^2*lambda_1*lambda_2 - A23*A24*B1_2*B1_4^2*lambda_1*lambda_3 - A23*A24*B1_2*B1_4^2*lambda_2*lambda_3 + A22*A43*B1_2*B1_4^2*lambda_1*lambda_2 + A23*A42*B1_2*B1_4^2*lambda_1*lambda_2 + A22*A43*B1_2*B1_4^2*lambda_1*lambda_3 + A23*A42*B1_2*B1_4^2*lambda_1*lambda_3 + A22*A43*B1_2*B1_4^2*lambda_2*lambda_3 + A23*A42*B1_2*B1_4^2*lambda_2*lambda_3 + A23*A44*B1_2^2*B1_4*lambda_1*lambda_2 + A24*A43*B1_2^2*B1_4*lambda_1*lambda_2 + A23*A44*B1_2^2*B1_4*lambda_1*lambda_3 + A24*A43*B1_2^2*B1_4*lambda_1*lambda_3 + A23*A44*B1_2^2*B1_4*lambda_2*lambda_3 + A24*A43*B1_2^2*B1_4*lambda_2*lambda_3 - A42*A43*B1_2^2*B1_4*lambda_1*lambda_2 - A42*A43*B1_2^2*B1_4*lambda_1*lambda_3 - A42*A43*B1_2^2*B1_4*lambda_2*lambda_3 + A42*A44*B1_2^3*lambda_1*lambda_2*lambda_3 - A23*B1_2*B1_4^2*lambda_1*lambda_2*lambda_3 + A43*B1_2^2*B1_4*lambda_1*lambda_2*lambda_3 + A22*A24*B1_2*B1_4^2*lambda_1*lambda_2*lambda_3 - 2*A22*A42*B1_2*B1_4^2*lambda_1*lambda_2*lambda_3 - A22*A44*B1_2^2*B1_4*lambda_1*lambda_2*lambda_3 - A24*A42*B1_2^2*B1_4*lambda_1*lambda_2*lambda_3))/((A23*B1_4 - A43*B1_2)*(A24^2*B1_2*B1_4^2 - 2*A24*A44*B1_2^2*B1_4 - A42*A24*B1_2*B1_4^2 + A22*A24*B1_4^3 + A44^2*B1_2^3 + A42*A44*B1_2^2*B1_4 - A22*A44*B1_2*B1_4^2 - A43*B1_2*B1_4^2 + A23*B1_4^3)), (1000000*(A23*A24^2*B1_4^3 - A43*A44^2*B1_2^3 + A23*B1_4^3*lambda_1*lambda_2 + A23*B1_4^3*lambda_1*lambda_3 + A23*B1_4^3*lambda_2*lambda_3 + A23*A44^2*B1_2^2*B1_4 - A24^2*A43*B1_2*B1_4^2 + A23*A24*B1_4^3*lambda_1 + A23*A24*B1_4^3*lambda_2 + A23*A24*B1_4^3*lambda_3 - 2*A23*A24*A44*B1_2*B1_4^2 + 2*A24*A43*A44*B1_2^2*B1_4 - A23*A44*B1_2*B1_4^2*lambda_1 - A24*A43*B1_2*B1_4^2*lambda_1 - A23*A44*B1_2*B1_4^2*lambda_2 - A24*A43*B1_2*B1_4^2*lambda_2 - A23*A44*B1_2*B1_4^2*lambda_3 - A24*A43*B1_2*B1_4^2*lambda_3 + A43*A44*B1_2^2*B1_4*lambda_1 + A43*A44*B1_2^2*B1_4*lambda_2 + A43*A44*B1_2^2*B1_4*lambda_3 - A43*B1_2*B1_4^2*lambda_1*lambda_2 - A43*B1_2*B1_4^2*lambda_1*lambda_3 - A43*B1_2*B1_4^2*lambda_2*lambda_3 - A22*B1_4^3*lambda_1*lambda_2*lambda_3 - A24*B1_2*B1_4^2*lambda_1*lambda_2*lambda_3 + A42*B1_2*B1_4^2*lambda_1*lambda_2*lambda_3 + A44*B1_2^2*B1_4*lambda_1*lambda_2*lambda_3))/((A23*B1_4 - A43*B1_2)*(A24^2*B1_2*B1_4^2 - 2*A24*A44*B1_2^2*B1_4 - A42*A24*B1_2*B1_4^2 + A22*A24*B1_4^3 + A44^2*B1_2^3 + A42*A44*B1_2^2*B1_4 - A22*A44*B1_2*B1_4^2 - A43*B1_2*B1_4^2 + A23*B1_4^3))];

%%%%%%%%%%%%%%%%%%%%%%%%%%%%%%%%%%%%%%%%%%%%%%%%%%%%%%%%%%%%%%%%%%%%%%%%%%%%

k_smc = 1000*1.5;   %10
sigma = 6000*1.5;    %60

sigma1 = S*X;

d_k = -(S*B1)\(S*A*X +S*L);
d_u = -(S*B1)\(n1*sigma*sqrt(abs(sigma1))*sign(sigma1) + Mu1);
dMu1 = -k_smc*sign(sigma1); 

ctrlVal = d_k + d_u;
U = real(ctrlVal);

== matlab function VehDynaPlayGround/Model helpers/Wrap2pi ==
  data: u input; y output
function y = wrapTo2Pi(u)

y = wrapTo2Pi(u);
